simulink model "VCU_SW"  (R2020b)
settings: Solver=FixedStepDiscrete  StartTime=0.0  StopTime=inf  FixedStep=1e-2  RelTol=1e-3
PreLoadFcn:
  | RTWConfigurationCB('preloadfcn', bdroot);
InitFcn:
  | loadvar_ttc500
undefined symbols (not defined in the file): BrkPedalTypes, CabMovModeTypes, cFuseTempSensAcc_X, cFuseTempSensAcc_Y, cFuseTempSensVal_X, cFuseTempSensVal_Y, cTMSTempSensVal_X, cTMSTempSensVal_Y, cTransferCaseSpeedRatio, diag_state, DoorsPositionTypes, dP_filter_Y, DriverOccClassSystemTypes, ErrorValueTypes, fatal_error_callback, IO_ADC_NO_RANGE, LadderStatusTypes, pAnalogCabRotSensAcc, pAnalogCabRotSensMaxVolt, pAnalogCabRotSensMinVolt, pAnalogCabRotSensRange, pAnalogCabRotSensZeroVolt, pBrkActivePress, pCabTiltSensAcc, pCabTiltSensMaxCur, pCabTiltSensMinCur, pDistanceCorrection, pECANManual_BPNEnable, pECANManual_BPNEnabler_Flag, pFilterSensAccRes, pHDirMaxDiffFrq, pHDirSensHighLvl, pHDirSensLowLvl, pMainGearRatio, pMaxFilterSensRes, pMaxFirstPedalSensValue, pMaxFuseTempSensRes, pMaxPressLoss, pMaxPressSensCurrent, pMaxPressValue, pMaxPressValueHydMotAndPump, pMaxPressValueParkDrain, pMaxSecondPedalSensValue, pMaxTempSensVoltage, pMaxTempValue, pMaxTMSTempSensRes, pMinFilterSensRes, pMinFirstPedalSensValue, pMinFuseTempSensRes, pMinPressLoss, pMinPressSensCurrent, pMinPressValue, pMinSecondPedalSensValue, pMinTempSensVoltage, pMinTempValue, pMinTMSTempSensRes, pMotorRingTeethNum, pPedalSensAccuracyPct, pPedalSensAccuracyVolt, pPressLossTreshhold ... (+20)
libraries: TTlibrary x270, canmsglib x127, simulink x88
(part 9 of 17)

== system VCU_SW/OutputLayer/OutputNetwork/OutputEngCAN/SetEngCAN50msec ==
  function : TriggerPort  TriggerType=function-call  VariantControl=Variant
  Bus Selector1 : BusSelector  OutputSignals=ID  OutputAsBus=on
  CANPack_VCU_ECU_TSC1 : canmsglib/CAN Pack  MsgList=(none)  MsgName=VCU_ECU_TSC1  MsgIDType=Extended (29-bit identifier)  MsgIdentifier=201326599  MsgLength=8  Remote=off  ApplyMinMax=off  BusOutput=on  SignalInfo={ 'VCU_ECU_TSC1_ContPurp', '35', '5', 'LE', 'unsigned', 'Standard', '0', '1', '0', '0', '31'; 'VCU_ECU_TSC1_EngOverContMod', '0', '2', 'LE', 'unsigned', 'Standard', '0', '1', '0', '0', '3'; 'VCU_ECU_TSC1_EngReqSpContCond', '2', '2', 'LE', 'unsigned', 'Standard', '0', '1', '0', '0', '3'; 'VCU_ECU_TSC1_EngReqSpSL', '8', '16', 'LE', 'unsigned', 'Standard', '0', '0.125', '0', '0', '8031.875'; 'VCU_ECU_TSC1_EngReqTrqHR', '40', '4', 'LE', 'unsigned', 'Standard', '0', '0.125', '0', '0', '0.875'; 'VCU_ECU_TSC1_EngReqTrqTL', '24', '8', 'LE', 'unsigned', 'Standard', '0', '1', '-125', '-125', '125'; 'VCU_ECU_TSC1_MesChksum', '60', '4', 'LE', 'unsigned', 'Standard', '0', '1', '0', '0', '15'; 'VCU_ECU_TSC1_MessCnt', '56', '4', 'LE', 'unsigned', 'Standard', '0', '1', '0', '0', '15'; 'VCU_ECU_TSC1_OverContModPr', '4', '2', 'LE', 'unsigned', 'Standard', '0', '1', '0', '0', '3'; 'VCU_ECU_TSC1_TransRate', '32', '3', 'LE', 'unsigned', 'Standard', '0', '1', '0', '0', '7' }
      settings: SourceProductBaseCode=ME,XP,VN  DataFormat=manually specified signals
  Constant1 : Constant  Value=uint8(0)
  Data Store Read1 : DataStoreRead  DataStoreName=OutputNetworkData  DataStoreElements=OutputNetworkData.EngCAN.ContPurp#OutputNetworkData.EngCAN.EngOverContMod#OutputNetworkData.EngCAN.EngReqSpContCond#OutputNetworkData.EngCAN.EngReqSpSL#OutputNetworkData.EngCAN.EngReqTrqHR#OutputNetworkData.EngCAN.EngReqTrqTL#OutputNetworkData.EngCAN.MesChksum#OutputNetworkData.EngCAN.MessCnt#OutputNetworkData.EngCAN.OverContModPr#OutputNetworkData.EngCAN.TransRate
  Function-Call Subsystem1 : Subsystem  TreatAsAtomicUnit=on
  Less Than1 : RelationalOperator  Operator=>  OutDataTypeStr=boolean  RndMeth=Simplest
  transmit_vcu_ecu_tsc1 : TTlibrary/CAN/transmit_message_name  channel=IO_CAN_CHANNEL_2  id_format=IO_CAN_EXT_FRAME  retranslation=off  io_error=on  sample_time=-1
      settings: SourceProductName=TT control 500 series
  wires:
  Less Than1/1 -> Function-Call Subsystem1/Enable
  Data Store Read1/2 -> CANPack_VCU_ECU_TSC1/2
  Data Store Read1/5 -> CANPack_VCU_ECU_TSC1/5
  Data Store Read1/1 -> CANPack_VCU_ECU_TSC1/1
  Constant1/1 -> Less Than1/2
  Data Store Read1/9 -> CANPack_VCU_ECU_TSC1/9
  Data Store Read1/8 -> CANPack_VCU_ECU_TSC1/8
  transmit_vcu_ecu_tsc1/1 -> Function-Call Subsystem1/2(error_sts), Less Than1/1  "error_tx_transmit_vcu_ecu_tsc1"
  Data Store Read1/6 -> CANPack_VCU_ECU_TSC1/6
  CANPack_VCU_ECU_TSC1/1 -> Bus Selector1/1, transmit_vcu_ecu_tsc1/1
  Data Store Read1/7 -> CANPack_VCU_ECU_TSC1/7
  Data Store Read1/10 -> CANPack_VCU_ECU_TSC1/10
  Data Store Read1/4 -> CANPack_VCU_ECU_TSC1/4
  Bus Selector1/1 -> Function-Call Subsystem1/1(In1)
  Data Store Read1/3 -> CANPack_VCU_ECU_TSC1/3

== system VCU_SW/OutputLayer/OutputNetwork/OutputHydCAN/SetHydCAN100msec ==
  note: См. outputFcn
  function : TriggerPort  TriggerType=function-call  VariantControl=Variant
  CANPack_hyd_Fluid_temp : canmsglib/CAN Pack  Commented=on  MsgList=(none)  MsgName=VEH_FLUID_TEMP  MsgIDType=Extended (29-bit identifier)  MsgIdentifier=419326202  MsgLength=1  Remote=off  ApplyMinMax=off  BusOutput=on  SignalInfo={ 'FluidTemp', '0', '8', 'LE', 'signed', 'Standard', '0', '1', '40', '-40', '120' }
      settings: SourceProductBaseCode=ME,XP,VN  DataFormat=manually specified signals
  Cabine1stLeftHydCylValve : Subsystem
  Cabine2ndRightHydCylValve : Subsystem
  CabineTurningValve : Subsystem
  Data Store Read : DataStoreRead  Commented=on  DataStoreName=OutputNetworkData  DataStoreElements=OutputNetworkData.HydCAN.fluidTemp
  Terminator : Terminator  Commented=on
  transmit_message_hyd_fluid_temp : TTlibrary/CAN/transmit_message_name  Commented=on  channel=IO_CAN_CHANNEL_0  id_format=IO_CAN_EXT_FRAME  retranslation=off  io_error=on  sample_time=-1
      settings: SourceProductName=TT control 500 series
  wires:
  transmit_message_hyd_fluid_temp/1 -> Terminator/1  "error_tx_transmit_message_hyd_fluid_temp"
  CANPack_hyd_Fluid_temp/1 -> transmit_message_hyd_fluid_temp/1
  Data Store Read/1 -> CANPack_hyd_Fluid_temp/1

== system VCU_SW/OutputLayer/OutputNetwork/OutputStrCAN/SetStrCAN100msec ==
  note: См. outputFcn
  function : TriggerPort  TriggerType=function-call  VariantControl=Variant
  CANPack_Str_Fluid_temp : canmsglib/CAN Pack  Commented=on  MsgList=(none)  MsgName=VEH_FLUID_TEMP  MsgIDType=Extended (29-bit identifier)  MsgIdentifier=419326202  MsgLength=1  Remote=off  ApplyMinMax=off  BusOutput=on  SignalInfo={ 'FluidTemp', '0', '8', 'LE', 'signed', 'Standard', '0', '1', '40', '-40', '120' }
      settings: SourceProductBaseCode=ME,XP,VN  DataFormat=manually specified signals
  CANPack_VLVCMD_STR1 : canmsglib/CAN Pack  MsgList=(none)  MsgName=VLVCMD_STR1  MsgIDType=Extended (29-bit identifier)  MsgIdentifier=217985274  MsgLength=3  Remote=off  ApplyMinMax=off  BusOutput=on  SignalInfo={ 'FailSafeModeCmdStr1', '22', '2', 'LE', 'unsigned', 'Standard', '0', '1', '0', '0', '3'; 'PortFlowCmdStr1', '0', '8', 'LE', 'unsigned', 'Standard', '0', '0.4', '0', '0', '100'; 'ValveStateStr1', '16', '4', 'LE', 'unsigned', 'Standard', '0', '1', '0', '0', '15' }
      settings: SourceProductBaseCode=ME,XP,VN  DataFormat=manually specified signals
  Data Store Read : DataStoreRead  Commented=on  DataStoreName=OutputNetworkData  DataStoreElements=OutputNetworkData.StrCAN.fluidTemp
  Data Store Read1 : DataStoreRead  DataStoreName=OutputNetworkData  DataStoreElements=OutputNetworkData.StrCAN.failSafeModeCmdStr1#OutputNetworkData.StrCAN.portFlowCmdStr1#OutputNetworkData.StrCAN.valveStateStr1
  Terminator : Terminator  Commented=on
  Terminator1 : Terminator
  transmit_message_str_fluid_temp : TTlibrary/CAN/transmit_message_name  Commented=on  channel=IO_CAN_CHANNEL_3  id_format=IO_CAN_EXT_FRAME  retranslation=off  io_error=on  sample_time=-1
      settings: SourceProductName=TT control 500 series
  transmit_message_vlvcmd_str1 : TTlibrary/CAN/transmit_message_name  channel=IO_CAN_CHANNEL_3  id_format=IO_CAN_EXT_FRAME  retranslation=off  io_error=on  sample_time=-1
      settings: SourceProductName=TT control 500 series
  wires:
  CANPack_Str_Fluid_temp/1 -> transmit_message_str_fluid_temp/1
  transmit_message_str_fluid_temp/1 -> Terminator/1  "error_tx_transmit_message_str_fluid_temp"
  Data Store Read/1 -> CANPack_Str_Fluid_temp/1
  Data Store Read1/1 -> CANPack_VLVCMD_STR1/1
  transmit_message_vlvcmd_str1/1 -> Terminator1/1  "error_tx_transmit_message_vlvcmd_str1"
  CANPack_VLVCMD_STR1/1 -> transmit_message_vlvcmd_str1/1
  Data Store Read1/2 -> CANPack_VLVCMD_STR1/2
  Data Store Read1/3 -> CANPack_VLVCMD_STR1/3

== system VCU_SW/logSignal/getListData/pageHighvoltageAppData/getListDataII1 ==
  getListDataII1 : TriggerPort  TriggerType=function-call  IsSimulinkFunction=on  FunctionName=getListDataII1  FunctionVisibility=scoped  VariantControl=(inherit)
  Constant : Constant  Value=uint8(5)
  Data Store Read1 : DataStoreRead  DataStoreName=sBmsCounter
  Data Store Read2 : DataStoreRead  DataStoreName=sChargeStopSignal
  Data Store Read3 : DataStoreRead  DataStoreName=sStopAll
  Data Store Read4 : DataStoreRead  DataStoreName=sBmsLocalState
  Demux11 : Demux  Outputs=2
  Function Caller : FunctionCaller  FunctionPrototype=data = getListData.splitIntoTwoBytes(value)  InputArgumentSpecifications=<Enter example>  OutputArgumentSpecifications=<Enter example>
  Ground : Ground
  Mux : Mux  Inputs=7
  data : ArgOut  DisableCoverage=on  OutDataTypeStr=uint8  PortDimensions=[1,7]  ArgumentName=data
  len : ArgOut  Port=2  OutDataTypeStr=uint8  ArgumentName=len
  wires:
  Data Store Read2/1 -> Mux/4
  Data Store Read3/1 -> Mux/5
  Demux11/2 -> Mux/3
  Data Store Read4/1 -> Mux/1
  Demux11/1 -> Mux/2
  Mux/1 -> data/1
  Constant/1 -> len/1
  Function Caller/1 -> Demux11/1
  Data Store Read1/1 -> Function Caller/1
  Ground/1 -> Mux/6, Mux/7

== system VCU_SW/logSignal/getListData/pageHighvoltageAppData/getListDataII10 ==
  getListDataII10 : TriggerPort  TriggerType=function-call  IsSimulinkFunction=on  FunctionName=getListDataII10  FunctionVisibility=scoped  VariantControl=(inherit)
  Constant : Constant  Value=uint8(4)
  Data Store Read1 : DataStoreRead  DataStoreName=sB5_modes_1
  Data Store Read2 : DataStoreRead  DataStoreName=sB5_mode_1
  Data Store Read5 : DataStoreRead  DataStoreName=sB5_ChargeMode
  Data Store Read6 : DataStoreRead  DataStoreName=sB5_power
  Ground : Ground
  Mux : Mux  Inputs=7
  data : ArgOut  DisableCoverage=on  OutDataTypeStr=uint8  PortDimensions=[1,7]  ArgumentName=data
  len : ArgOut  Port=2  OutDataTypeStr=uint8  ArgumentName=len
  wires:
  Mux/1 -> data/1
  Constant/1 -> len/1
  Data Store Read5/1 -> Mux/4
  Data Store Read6/1 -> Mux/3
  Data Store Read2/1 -> Mux/1
  Data Store Read1/1 -> Mux/2
  Ground/1 -> Mux/7, Mux/6, Mux/5

== system VCU_SW/logSignal/getListData/pageHighvoltageAppData/getListDataII11 ==
  getListDataII11 : TriggerPort  TriggerType=function-call  IsSimulinkFunction=on  FunctionName=getListDataII11  FunctionVisibility=scoped  VariantControl=(inherit)
  Constant : Constant  Value=uint8(5)
  Data Store Read1 : DataStoreRead  DataStoreName=sPlugUnlockPerm
  Data Store Read2 : DataStoreRead  DataStoreName=sChargeLocalState
  Data Store Read3 : DataStoreRead  DataStoreName=sChargePerm
  Data Store Read4 : DataStoreRead  DataStoreName=sPlugLockPerm
  Data Store Read5 : DataStoreRead  DataStoreName=sPrechargeComplete
  Ground : Ground
  Mux : Mux  Inputs=7
  data : ArgOut  DisableCoverage=on  OutDataTypeStr=uint8  PortDimensions=[1,7]  ArgumentName=data
  len : ArgOut  Port=2  OutDataTypeStr=uint8  ArgumentName=len
  wires:
  Mux/1 -> data/1
  Constant/1 -> len/1
  Data Store Read4/1 -> Mux/1
  Data Store Read1/1 -> Mux/2
  Data Store Read3/1 -> Mux/3
  Data Store Read2/1 -> Mux/4
  Data Store Read5/1 -> Mux/5
  Ground/1 -> Mux/6, Mux/7

== system VCU_SW/logSignal/getListData/pageHighvoltageAppData/getListDataII12 ==
  note: -32767 to 32767
  getListDataII12 : TriggerPort  TriggerType=function-call  IsSimulinkFunction=on  FunctionName=getListDataII12  FunctionVisibility=scoped  VariantControl=(inherit)
  Constant : Constant  Value=uint8(6)
  Data Store Read1 : DataStoreRead  DataStoreName=sAimTrq
  Data Store Read2 : DataStoreRead  DataStoreName=sT15GroupStt
  Data Store Read4 : DataStoreRead  DataStoreName=sInvLocalState
  Data Store Read5 : DataStoreRead  DataStoreName=sCurStepInv
  Data Type Conversion : DataTypeConversion  OutDataTypeStr=int32
  Data Type Conversion1 : DataTypeConversion  OutDataTypeStr=uint16
  Data Type Conversion2 : DataTypeConversion  OutDataTypeStr=int32
  Data Type Conversion3 : DataTypeConversion  OutDataTypeStr=uint16
  Demux1 : Demux  Outputs=2
  Demux11 : Demux  Outputs=2
  Function Caller : FunctionCaller  FunctionPrototype=data = getListData.splitIntoTwoBytes(value)  InputArgumentSpecifications=<Enter example>  OutputArgumentSpecifications=<Enter example>
  Function Caller1 : FunctionCaller  FunctionPrototype=data = getListData.splitIntoTwoBytes(value)  InputArgumentSpecifications=<Enter example>  OutputArgumentSpecifications=<Enter example>
  Ground : Ground
  Mux : Mux  Inputs=7
  Sum2 : Sum  Inputs=++|
  Sum3 : Sum  Inputs=|++
  offset : Constant  Value=int32(32767)
  data : ArgOut  DisableCoverage=on  OutDataTypeStr=uint8  PortDimensions=[1,7]  ArgumentName=data
  len : ArgOut  Port=2  OutDataTypeStr=uint8  ArgumentName=len
  wires:
  Ground/1 -> Mux/7
  Constant/1 -> len/1
  Mux/1 -> data/1
  Demux11/2 -> Mux/3
  Data Store Read1/1 -> Data Type Conversion2/1
  Function Caller/1 -> Demux11/1
  Demux11/1 -> Mux/2
  Data Store Read4/1 -> Mux/1
  Function Caller1/1 -> Demux1/1
  Demux1/2 -> Mux/5
  Demux1/1 -> Mux/4
  Data Store Read2/1 -> Mux/6
  Data Store Read5/1 -> Data Type Conversion/1
  Sum2/1 -> Data Type Conversion1/1
  Data Type Conversion1/1 -> Function Caller1/1
  Data Type Conversion/1 -> Sum2/2
  offset/1 -> Sum2/1, Sum3/2
  Sum3/1 -> Data Type Conversion3/1
  Data Type Conversion2/1 -> Sum3/1
  Data Type Conversion3/1 -> Function Caller/1

== system VCU_SW/logSignal/getListData/pageHighvoltageAppData/getListDataII2 ==
  getListDataII2 : TriggerPort  TriggerType=function-call  IsSimulinkFunction=on  FunctionName=getListDataII2  FunctionVisibility=scoped  VariantControl=(inherit)
  Constant : Constant  Value=uint8(4)
  Data Store Read1 : DataStoreRead  DataStoreName=sPermissibleChargeCurrent
  Data Store Read2 : DataStoreRead  DataStoreName=sPermissibleChargeVoltage
  Demux1 : Demux  Outputs=2
  Demux11 : Demux  Outputs=2
  Function Caller : FunctionCaller  FunctionPrototype=data = getListData.splitIntoTwoBytes(value)  InputArgumentSpecifications=<Enter example>  OutputArgumentSpecifications=<Enter example>
  Function Caller1 : FunctionCaller  FunctionPrototype=data = getListData.splitIntoTwoBytes(value)  InputArgumentSpecifications=<Enter example>  OutputArgumentSpecifications=<Enter example>
  Ground : Ground
  Mux : Mux  Inputs=7
  data : ArgOut  DisableCoverage=on  OutDataTypeStr=uint8  PortDimensions=[1,7]  ArgumentName=data
  len : ArgOut  Port=2  OutDataTypeStr=uint8  ArgumentName=len
  wires:
  Mux/1 -> data/1
  Constant/1 -> len/1
  Function Caller/1 -> Demux11/1
  Demux11/1 -> Mux/1
  Data Store Read1/1 -> Function Caller/1
  Demux11/2 -> Mux/2
  Demux1/1 -> Mux/3
  Function Caller1/1 -> Demux1/1
  Data Store Read2/1 -> Function Caller1/1
  Demux1/2 -> Mux/4
  Ground/1 -> Mux/5, Mux/6, Mux/7

== system VCU_SW/logSignal/getListData/pageHighvoltageAppData/getListDataII3 ==
  getListDataII3 : TriggerPort  TriggerType=function-call  IsSimulinkFunction=on  FunctionName=getListDataII3  FunctionVisibility=scoped  VariantControl=(inherit)
  Constant : Constant  Value=uint8(7)
  Data Store Read1 : DataStoreRead  DataStoreName=sCompressorPwm
  Data Store Read2 : DataStoreRead  DataStoreName=sTmsCounter
  Data Store Read3 : DataStoreRead  DataStoreName=sPumpPwm
  Data Store Read4 : DataStoreRead  DataStoreName=sFanControl
  Data Store Read5 : DataStoreRead  DataStoreName=sTmsLocalState
  Data Store Read6 : DataStoreRead  DataStoreName=sTmsCircleSelected
  Demux1 : Demux  Outputs=2
  Function Caller1 : FunctionCaller  FunctionPrototype=data = getListData.splitIntoTwoBytes(value)  InputArgumentSpecifications=<Enter example>  OutputArgumentSpecifications=<Enter example>
  Mux : Mux  Inputs=7
  data : ArgOut  DisableCoverage=on  OutDataTypeStr=uint8  PortDimensions=[1,7]  ArgumentName=data
  len : ArgOut  Port=2  OutDataTypeStr=uint8  ArgumentName=len
  wires:
  Mux/1 -> data/1
  Constant/1 -> len/1
  Function Caller1/1 -> Demux1/1
  Data Store Read2/1 -> Function Caller1/1
  Demux1/1 -> Mux/6
  Demux1/2 -> Mux/7
  Data Store Read1/1 -> Mux/1
  Data Store Read3/1 -> Mux/2
  Data Store Read4/1 -> Mux/3
  Data Store Read5/1 -> Mux/4
  Data Store Read6/1 -> Mux/5

== system VCU_SW/logSignal/getListData/pageHighvoltageAppData/getListDataII4 ==
  getListDataII4 : TriggerPort  TriggerType=function-call  IsSimulinkFunction=on  FunctionName=getListDataII4  FunctionVisibility=scoped  VariantControl=(inherit)
  Constant : Constant  Value=uint8(7)
  Data Store Read1 : DataStoreRead  DataStoreName=sCompressorCounter
  Data Store Read2 : DataStoreRead  DataStoreName=sValveControl
  Data Store Read3 : DataStoreRead  DataStoreName=sPreviousState
  Data Store Read4 : DataStoreRead  DataStoreName=sHeaterEnable
  Data Store Read5 : DataStoreRead  DataStoreName=sHeaterPowerControl
  Data Store Read6 : DataStoreRead  DataStoreName=sCompressorStart
  Demux11 : Demux  Outputs=2
  Function Caller : FunctionCaller  FunctionPrototype=data = getListData.splitIntoTwoBytes(value)  InputArgumentSpecifications=<Enter example>  OutputArgumentSpecifications=<Enter example>
  Mux : Mux  Inputs=7
  data : ArgOut  DisableCoverage=on  OutDataTypeStr=uint8  PortDimensions=[1,7]  ArgumentName=data
  len : ArgOut  Port=2  OutDataTypeStr=uint8  ArgumentName=len
  wires:
  Mux/1 -> data/1
  Constant/1 -> len/1
  Function Caller/1 -> Demux11/1
  Demux11/1 -> Mux/1
  Data Store Read1/1 -> Function Caller/1
  Demux11/2 -> Mux/2
  Data Store Read3/1 -> Mux/6
  Data Store Read2/1 -> Mux/7
  Data Store Read4/1 -> Mux/5
  Data Store Read5/1 -> Mux/4
  Data Store Read6/1 -> Mux/3

== system VCU_SW/logSignal/getListData/pageHighvoltageAppData/getListDataII5 ==
  getListDataII5 : TriggerPort  TriggerType=function-call  IsSimulinkFunction=on  FunctionName=getListDataII5  FunctionVisibility=scoped  VariantControl=(inherit)
  Constant : Constant  Value=uint8(7)
  Data Store Read1 : DataStoreRead  DataStoreName=sSelfCircCounter
  Data Store Read2 : DataStoreRead  DataStoreName=sCompressoSecondCircleEx
  Data Store Read3 : DataStoreRead  DataStoreName=sCompressorStartEx
  Data Store Read4 : DataStoreRead  DataStoreName=sCompressorOffEx
  Data Store Read5 : DataStoreRead  DataStoreName=sPumpSecondCircleEx
  Data Store Read6 : DataStoreRead  DataStoreName=sPumpOffEx
  Demux11 : Demux  Outputs=2
  Function Caller : FunctionCaller  FunctionPrototype=data = getListData.splitIntoTwoBytes(value)  InputArgumentSpecifications=<Enter example>  OutputArgumentSpecifications=<Enter example>
  Mux : Mux  Inputs=7
  data : ArgOut  DisableCoverage=on  OutDataTypeStr=uint8  PortDimensions=[1,7]  ArgumentName=data
  len : ArgOut  Port=2  OutDataTypeStr=uint8  ArgumentName=len
  wires:
  Mux/1 -> data/1
  Constant/1 -> len/1
  Function Caller/1 -> Demux11/1
  Demux11/1 -> Mux/1
  Data Store Read1/1 -> Function Caller/1
  Demux11/2 -> Mux/2
  Data Store Read2/1 -> Mux/7
  Data Store Read3/1 -> Mux/6
  Data Store Read4/1 -> Mux/5
  Data Store Read5/1 -> Mux/4
  Data Store Read6/1 -> Mux/3

== system VCU_SW/logSignal/getListData/pageHighvoltageAppData/getListDataII6 ==
  getListDataII6 : TriggerPort  TriggerType=function-call  IsSimulinkFunction=on  FunctionName=getListDataII6  FunctionVisibility=scoped  VariantControl=(inherit)
  Constant : Constant  Value=uint8(7)
  Data Store Read1 : DataStoreRead  DataStoreName=sEproCurrent
  Data Store Read2 : DataStoreRead  DataStoreName=sHeaterSecondCircleEx
  Data Store Read3 : DataStoreRead  DataStoreName=sHeaterTempEx
  Data Store Read4 : DataStoreRead  DataStoreName=sHeaterOffEx
  Data Store Read5 : DataStoreRead  DataStoreName=sEproStartCommand
  Data Store Read6 : DataStoreRead  DataStoreName=sEproPower
  Demux11 : Demux  Outputs=2
  Function Caller : FunctionCaller  FunctionPrototype=data = getListData.splitIntoTwoBytes(value)  InputArgumentSpecifications=<Enter example>  OutputArgumentSpecifications=<Enter example>
  Mux : Mux  Inputs=7
  data : ArgOut  DisableCoverage=on  OutDataTypeStr=uint8  PortDimensions=[1,7]  ArgumentName=data
  len : ArgOut  Port=2  OutDataTypeStr=uint8  ArgumentName=len
  wires:
  Mux/1 -> data/1
  Constant/1 -> len/1
  Data Store Read3/1 -> Mux/2
  Data Store Read4/1 -> Mux/1
  Data Store Read2/1 -> Mux/3
  Demux11/2 -> Mux/6
  Data Store Read1/1 -> Function Caller/1
  Function Caller/1 -> Demux11/1
  Demux11/1 -> Mux/5
  Data Store Read5/1 -> Mux/7
  Data Store Read6/1 -> Mux/4

== system VCU_SW/logSignal/getListData/pageHighvoltageAppData/getListDataII7 ==
  getListDataII7 : TriggerPort  TriggerType=function-call  IsSimulinkFunction=on  FunctionName=getListDataII7  FunctionVisibility=scoped  VariantControl=(inherit)
  Constant : Constant  Value=uint8(6)
  Data Store Read1 : DataStoreRead  DataStoreName=sPosIsolationResistence
  Data Store Read2 : DataStoreRead  DataStoreName=sNegIsolationResistence
  Data Store Read3 : DataStoreRead  DataStoreName=sMaxCellVoltage
  Demux1 : Demux  Outputs=2
  Demux11 : Demux  Outputs=2
  Demux2 : Demux  Outputs=2
  Function Caller : FunctionCaller  FunctionPrototype=data = getListData.splitIntoTwoBytes(value)  InputArgumentSpecifications=<Enter example>  OutputArgumentSpecifications=<Enter example>
  Function Caller1 : FunctionCaller  FunctionPrototype=data = getListData.splitIntoTwoBytes(value)  InputArgumentSpecifications=<Enter example>  OutputArgumentSpecifications=<Enter example>
  Function Caller2 : FunctionCaller  FunctionPrototype=data = getListData.splitIntoTwoBytes(value)  InputArgumentSpecifications=<Enter example>  OutputArgumentSpecifications=<Enter example>
  Ground : Ground
  Mux : Mux  Inputs=7
  data : ArgOut  DisableCoverage=on  OutDataTypeStr=uint8  PortDimensions=[1,7]  ArgumentName=data
  len : ArgOut  Port=2  OutDataTypeStr=uint8  ArgumentName=len
  wires:
  Demux11/2 -> Mux/2
  Data Store Read1/1 -> Function Caller/1
  Demux11/1 -> Mux/1
  Function Caller/1 -> Demux11/1
  Constant/1 -> len/1
  Mux/1 -> data/1
  Function Caller1/1 -> Demux1/1
  Demux1/1 -> Mux/3
  Data Store Read2/1 -> Function Caller1/1
  Demux1/2 -> Mux/4
  Demux2/2 -> Mux/6
  Data Store Read3/1 -> Function Caller2/1
  Demux2/1 -> Mux/5
  Function Caller2/1 -> Demux2/1
  Ground/1 -> Mux/7

== system VCU_SW/logSignal/getListData/pageHighvoltageAppData/getListDataII8 ==
  getListDataII8 : TriggerPort  TriggerType=function-call  IsSimulinkFunction=on  FunctionName=getListDataII8  FunctionVisibility=scoped  VariantControl=(inherit)
  Constant : Constant  Value=uint8(6)
  Data Store Read1 : DataStoreRead  DataStoreName=sMinCellVoltage
  Data Store Read2 : DataStoreRead  DataStoreName=sMaxBatTemp
  Data Store Read3 : DataStoreRead  DataStoreName=sMinBatTemp
  Demux1 : Demux  Outputs=2
  Demux11 : Demux  Outputs=2
  Demux2 : Demux  Outputs=2
  Function Caller : FunctionCaller  FunctionPrototype=data = getListData.splitIntoTwoBytes(value)  InputArgumentSpecifications=<Enter example>  OutputArgumentSpecifications=<Enter example>
  Function Caller1 : FunctionCaller  FunctionPrototype=data = getListData.splitIntoTwoBytes(value)  InputArgumentSpecifications=<Enter example>  OutputArgumentSpecifications=<Enter example>
  Function Caller2 : FunctionCaller  FunctionPrototype=data = getListData.splitIntoTwoBytes(value)  InputArgumentSpecifications=<Enter example>  OutputArgumentSpecifications=<Enter example>
  Ground : Ground
  Mux : Mux  Inputs=7
  data : ArgOut  DisableCoverage=on  OutDataTypeStr=uint8  PortDimensions=[1,7]  ArgumentName=data
  len : ArgOut  Port=2  OutDataTypeStr=uint8  ArgumentName=len
  wires:
  Mux/1 -> data/1
  Constant/1 -> len/1
  Function Caller/1 -> Demux11/1
  Demux11/1 -> Mux/1
  Data Store Read1/1 -> Function Caller/1
  Demux11/2 -> Mux/2
  Demux1/2 -> Mux/4
  Data Store Read2/1 -> Function Caller1/1
  Demux1/1 -> Mux/3
  Function Caller1/1 -> Demux1/1
  Function Caller2/1 -> Demux2/1
  Demux2/2 -> Mux/6
  Demux2/1 -> Mux/5
  Ground/1 -> Mux/7
  Data Store Read3/1 -> Function Caller2/1

== system VCU_SW/logSignal/getListData/pageHighvoltageAppData/getListDataII9 ==
  getListDataII9 : TriggerPort  TriggerType=function-call  IsSimulinkFunction=on  FunctionName=getListDataII9  FunctionVisibility=scoped  VariantControl=(inherit)
  Constant : Constant  Value=uint8(6)
  Data Store Read1 : DataStoreRead  DataStoreName=sTotalVoltage
  Data Store Read2 : DataStoreRead  DataStoreName=sMaxCellVoltTemp
  Data Store Read3 : DataStoreRead  DataStoreName=sMinCellVoltTemp
  Data Store Read4 : DataStoreRead  DataStoreName=sSettingTargetWaterTemp
  Data Store Read5 : DataStoreRead  DataStoreName=sAverageBatTemp
  Demux11 : Demux  Outputs=2
  Function Caller : FunctionCaller  FunctionPrototype=data = getListData.splitIntoTwoBytes(value)  InputArgumentSpecifications=<Enter example>  OutputArgumentSpecifications=<Enter example>
  Ground : Ground
  Mux : Mux  Inputs=7
  data : ArgOut  DisableCoverage=on  OutDataTypeStr=uint8  PortDimensions=[1,7]  ArgumentName=data
  len : ArgOut  Port=2  OutDataTypeStr=uint8  ArgumentName=len
  wires:
  Data Store Read1/1 -> Function Caller/1
  Function Caller/1 -> Demux11/1
  Constant/1 -> len/1
  Mux/1 -> data/1
  Demux11/1 -> Mux/3
  Demux11/2 -> Mux/4
  Data Store Read3/1 -> Mux/2
  Data Store Read2/1 -> Mux/1
  Data Store Read4/1 -> Mux/5
  Data Store Read5/1 -> Mux/6
  Ground/1 -> Mux/7

== system VCU_SW/logSignal/getListData/pageOutputRawData/getListDataOI1 ==
  getListDataOI1 : TriggerPort  TriggerType=function-call  IsSimulinkFunction=on  FunctionName=getListDataOI1  FunctionVisibility=scoped  VariantControl=(inherit)
  Data Store Read2 : DataStoreRead  DataStoreName=sCoolSensSup
  Data Store Read3 : DataStoreRead  DataStoreName=sOnBrdChrgTermSttSup
  Data Store Read4 : DataStoreRead  DataStoreName=sHVILSup
  Data Store Read5 : DataStoreRead  DataStoreName=sOnBrdFastChrgSup
  Data Store Read6 : DataStoreRead  DataStoreName=sPressSensSup
  Data Store Read7 : DataStoreRead  DataStoreName=sGearboxSensSup
  Data Store Read8 : DataStoreRead  DataStoreName=sACDCChrgConvSwt
  Mux : Mux  Inputs=7
  data : ArgOut  DisableCoverage=on  OutDataTypeStr=uint8  PortDimensions=[1,7]  ArgumentName=data
  wires:
  Mux/1 -> data/1
  Data Store Read2/1 -> Mux/7
  Data Store Read3/1 -> Mux/6
  Data Store Read8/1 -> Mux/1
  Data Store Read4/1 -> Mux/5
  Data Store Read7/1 -> Mux/2
  Data Store Read5/1 -> Mux/4
  Data Store Read6/1 -> Mux/3

== system VCU_SW/logSignal/getListData/pageOutputRawData/getListDataOI2 ==
  getListDataOI2 : TriggerPort  TriggerType=function-call  IsSimulinkFunction=on  FunctionName=getListDataOI2  FunctionVisibility=scoped  VariantControl=(inherit)
  Data Store Read : DataStoreRead  DataStoreName=sCapsSup
  Data Store Read1 : DataStoreRead  DataStoreName=sPumpFlowSetPnt
  Data Store Read12 : DataStoreRead  DataStoreName=sTMSComprSetPnt
  Data Store Read13 : DataStoreRead  DataStoreName=sCircPumpSetPnt
  Demux : Demux  Outputs=2
  Demux1 : Demux  Outputs=2
  Demux2 : Demux  Outputs=2
  Function Caller3 : FunctionCaller  FunctionPrototype=data = getListData.splitIntoTwoBytes(value)  InputArgumentSpecifications=<Enter example>  OutputArgumentSpecifications=<Enter example>
  Function Caller4 : FunctionCaller  FunctionPrototype=data = getListData.splitIntoTwoBytes(value)  InputArgumentSpecifications=<Enter example>  OutputArgumentSpecifications=<Enter example>
  Function Caller5 : FunctionCaller  FunctionPrototype=data = getListData.splitIntoTwoBytes(value)  InputArgumentSpecifications=<Enter example>  OutputArgumentSpecifications=<Enter example>
  Mux1 : Mux  Inputs=7
  data : ArgOut  DisableCoverage=on  OutDataTypeStr=uint8  PortDimensions=[1,7]  ArgumentName=data
  wires:
  Mux1/1 -> data/1
  Data Store Read12/1 -> Function Caller4/1
  Demux1/1 -> Mux1/3
  Demux/2 -> Mux1/2
  Demux2/1 -> Mux1/5
  Demux/1 -> Mux1/1
  Data Store Read13/1 -> Function Caller5/1
  Demux2/2 -> Mux1/6
  Function Caller3/1 -> Demux/1
  Data Store Read1/1 -> Function Caller3/1
  Data Store Read/1 -> Mux1/7
  Demux1/2 -> Mux1/4
  Function Caller4/1 -> Demux1/1
  Function Caller5/1 -> Demux2/1

== system VCU_SW/logSignal/getListData/pageOutputRawData/getListDataOI3 ==
  getListDataOI3 : TriggerPort  TriggerType=function-call  IsSimulinkFunction=on  FunctionName=getListDataOI3  FunctionVisibility=scoped  VariantControl=(inherit)
  Data Store Read10 : DataStoreRead  DataStoreName=sSecondGearVlvSetPnt
  Data Store Read11 : DataStoreRead  DataStoreName=sRemBrkVlvSetPnt
  Data Store Read9 : DataStoreRead  DataStoreName=sFirstGearVlvSetPnt
  Demux3 : Demux  Outputs=2
  Demux4 : Demux  Outputs=2
  Demux5 : Demux  Outputs=2
  Function Caller : FunctionCaller  FunctionPrototype=data = getListData.splitIntoTwoBytes(value)  InputArgumentSpecifications=<Enter example>  OutputArgumentSpecifications=<Enter example>
  Function Caller1 : FunctionCaller  FunctionPrototype=data = getListData.splitIntoTwoBytes(value)  InputArgumentSpecifications=<Enter example>  OutputArgumentSpecifications=<Enter example>
  Function Caller2 : FunctionCaller  FunctionPrototype=data = getListData.splitIntoTwoBytes(value)  InputArgumentSpecifications=<Enter example>  OutputArgumentSpecifications=<Enter example>
  Ground : Ground
  Mux2 : Mux  Inputs=7
  data : ArgOut  DisableCoverage=on  OutDataTypeStr=uint8  PortDimensions=[1,7]  ArgumentName=data
  wires:
  Function Caller1/1 -> Demux4/1
  Function Caller2/1 -> Demux5/1
  Demux4/2 -> Mux2/4
  Demux3/2 -> Mux2/2
  Demux5/1 -> Mux2/5
  Demux3/1 -> Mux2/1
  Demux4/1 -> Mux2/3
  Data Store Read9/1 -> Function Caller/1
  Data Store Read10/1 -> Function Caller1/1
  Ground/1 -> Mux2/7
  Function Caller/1 -> Demux3/1
  Demux5/2 -> Mux2/6
  Data Store Read11/1 -> Function Caller2/1
  Mux2/1 -> data/1

== system VCU_SW/logSignal/getListData/pageRawInput/getListDataII1 ==
  getListDataII1 : TriggerPort  TriggerType=function-call  IsSimulinkFunction=on  FunctionName=getListDataII1  FunctionVisibility=scoped  VariantControl=(inherit)
  Constant : Constant  Value=uint8(7)
  Data Store Read1 : DataStoreRead  DataStoreName=sHVILSup
  Data Store Read2 : DataStoreRead  DataStoreName=sPrechargeCtrlStt
  Data Store Read3 : DataStoreRead  DataStoreName=sDCDCEmergGND
  Data Store Read4 : DataStoreRead  DataStoreName=sACChrgSupTermStt
  Data Store Read5 : DataStoreRead  DataStoreName=sACChrgGndTermStt
  Data Store Read6 : DataStoreRead  DataStoreName=sDCChrgSupTermStt
  Data Store Read7 : DataStoreRead  DataStoreName=sDCChrgGndTermStt
  Mux : Mux  Inputs=7
  data : ArgOut  DisableCoverage=on  OutDataTypeStr=uint8  PortDimensions=[1,7]  ArgumentName=data
  len : ArgOut  Port=2  OutDataTypeStr=uint8  ArgumentName=len
  wires:
  Data Store Read5/1 -> Mux/4
  Data Store Read2/1 -> Mux/7
  Data Store Read3/1 -> Mux/5
  Data Store Read7/1 -> Mux/3
  Data Store Read4/1 -> Mux/1
  Data Store Read6/1 -> Mux/2
  Data Store Read1/1 -> Mux/6
  Mux/1 -> data/1
  Constant/1 -> len/1

== system VCU_SW/logSignal/getListData/pageRawInput/getListDataII2 ==
  getListDataII2 : TriggerPort  TriggerType=function-call  IsSimulinkFunction=on  FunctionName=getListDataII2  FunctionVisibility=scoped  VariantControl=(inherit)
  Constant : Constant  Value=uint8(7)
  Data Store Read : DataStoreRead  DataStoreName=sGlobalSupTermStt
  Data Store Read10 : DataStoreRead  DataStoreName=sFrontCargoWeight
  Data Store Read11 : DataStoreRead  DataStoreName=sRearCargoWeight
  Data Store Read14 : DataStoreRead  DataStoreName=sGearboxOilState
  Demux : Demux  Outputs=2
  Demux1 : Demux  Outputs=2
  Demux2 : Demux  Outputs=2
  Function Caller : FunctionCaller  FunctionPrototype=data = getListData.splitIntoTwoBytes(value)  InputArgumentSpecifications=<Enter example>  OutputArgumentSpecifications=<Enter example>
  Function Caller13 : FunctionCaller  FunctionPrototype=data = getListData.splitIntoTwoBytes(value)  InputArgumentSpecifications=<Enter example>  OutputArgumentSpecifications=<Enter example>
  Function Caller14 : FunctionCaller  FunctionPrototype=data = getListData.splitIntoTwoBytes(value)  InputArgumentSpecifications=<Enter example>  OutputArgumentSpecifications=<Enter example>
  Mux1 : Mux  Inputs=7
  data : ArgOut  DisableCoverage=on  OutDataTypeStr=uint8  PortDimensions=[1,7]  ArgumentName=data
  len : ArgOut  Port=2  OutDataTypeStr=uint8  ArgumentName=len
  wires:
  Data Store Read/1 -> Mux1/7
  Data Store Read14/1 -> Function Caller/1
  Demux2/2 -> Mux1/6
  Demux2/1 -> Mux1/5
  Demux/2 -> Mux1/2
  Data Store Read10/1 -> Function Caller13/1
  Demux/1 -> Mux1/1
  Function Caller/1 -> Demux/1
  Function Caller13/1 -> Demux1/1
  Demux1/1 -> Mux1/3
  Demux1/2 -> Mux1/4
  Function Caller14/1 -> Demux2/1
  Data Store Read11/1 -> Function Caller14/1
  Mux1/1 -> data/1
  Constant/1 -> len/1

== system VCU_SW/logSignal/getListData/pageRawInput/getListDataII3 ==
  getListDataII3 : TriggerPort  TriggerType=function-call  IsSimulinkFunction=on  FunctionName=getListDataII3  FunctionVisibility=scoped  VariantControl=(inherit)
  Constant : Constant  Value=uint8(6)
  Data Store Read12 : DataStoreRead  DataStoreName=sTMSTempInput
  Data Store Read17 : DataStoreRead  DataStoreName=sPumpFlowCur
  Demux3 : Demux
  Demux4 : Demux  Outputs=2
  Function Caller1 : FunctionCaller  FunctionPrototype=data = getListData.splitIntoFourBytes(value)  InputArgumentSpecifications=<Enter example>  OutputArgumentSpecifications=<Enter example>
  Function Caller2 : FunctionCaller  FunctionPrototype=data = getListData.splitIntoTwoBytes(value)  InputArgumentSpecifications=<Enter example>  OutputArgumentSpecifications=<Enter example>
  Ground : Ground
  Mux2 : Mux  Inputs=7
  data : ArgOut  DisableCoverage=on  OutDataTypeStr=uint8  PortDimensions=[1,7]  ArgumentName=data
  len : ArgOut  Port=2  OutDataTypeStr=uint8  ArgumentName=len
  wires:
  Demux4/2 -> Mux2/6
  Ground/1 -> Mux2/7
  Demux3/4 -> Mux2/4
  Demux3/2 -> Mux2/2
  Function Caller2/1 -> Demux4/1
  Data Store Read17/1 -> Function Caller2/1
  Demux3/1 -> Mux2/1
  Demux4/1 -> Mux2/5
  Function Caller1/1 -> Demux3/1
  Data Store Read12/1 -> Function Caller1/1
  Demux3/3 -> Mux2/3
  Mux2/1 -> data/1
  Constant/1 -> len/1

== system VCU_SW/logSignal/getListData/pageRawInput/getListDataII4 ==
  getListDataII4 : TriggerPort  TriggerType=function-call  IsSimulinkFunction=on  FunctionName=getListDataII4  FunctionVisibility=scoped  VariantControl=(inherit)
  Constant : Constant  Value=uint8(6)
  Data Store Read13 : DataStoreRead  DataStoreName=sTMSTempOutput
  Data Store Read18 : DataStoreRead  DataStoreName=sFirstGearVlvCur
  Demux5 : Demux
  Demux6 : Demux  Outputs=2
  Function Caller3 : FunctionCaller  FunctionPrototype=data = getListData.splitIntoTwoBytes(value)  InputArgumentSpecifications=<Enter example>  OutputArgumentSpecifications=<Enter example>
  Function Caller8 : FunctionCaller  FunctionPrototype=data = getListData.splitIntoFourBytes(value)  InputArgumentSpecifications=<Enter example>  OutputArgumentSpecifications=<Enter example>
  Ground1 : Ground
  Mux3 : Mux  Inputs=7
  data : ArgOut  DisableCoverage=on  OutDataTypeStr=uint8  PortDimensions=[1,7]  ArgumentName=data
  len : ArgOut  Port=2  OutDataTypeStr=uint8  ArgumentName=len
  wires:
  Function Caller8/1 -> Demux5/1
  Function Caller3/1 -> Demux6/1
  Data Store Read13/1 -> Function Caller8/1
  Demux6/2 -> Mux3/6
  Demux6/1 -> Mux3/5
  Data Store Read18/1 -> Function Caller3/1
  Demux5/2 -> Mux3/2
  Demux5/3 -> Mux3/3
  Demux5/4 -> Mux3/4
  Demux5/1 -> Mux3/1
  Ground1/1 -> Mux3/7
  Mux3/1 -> data/1
  Constant/1 -> len/1

== system VCU_SW/logSignal/getListData/pageRawInput/getListDataII5 ==
  getListDataII5 : TriggerPort  TriggerType=function-call  IsSimulinkFunction=on  FunctionName=getListDataII5  FunctionVisibility=scoped  VariantControl=(inherit)
  Constant : Constant  Value=uint8(6)
  Data Store Read19 : DataStoreRead  DataStoreName=sSecondGearVlvCur
  Data Store Read8 : DataStoreRead  DataStoreName=sFuseBoxTempSens1
  Demux7 : Demux
  Demux8 : Demux  Outputs=2
  Function Caller4 : FunctionCaller  FunctionPrototype=data = getListData.splitIntoTwoBytes(value)  InputArgumentSpecifications=<Enter example>  OutputArgumentSpecifications=<Enter example>
  Function Caller9 : FunctionCaller  FunctionPrototype=data = getListData.splitIntoFourBytes(value)  InputArgumentSpecifications=<Enter example>  OutputArgumentSpecifications=<Enter example>
  Ground2 : Ground
  Mux4 : Mux  Inputs=7
  data : ArgOut  DisableCoverage=on  OutDataTypeStr=uint8  PortDimensions=[1,7]  ArgumentName=data
  len : ArgOut  Port=2  OutDataTypeStr=uint8  ArgumentName=len
  wires:
  Function Caller9/1 -> Demux7/1
  Data Store Read19/1 -> Function Caller4/1
  Ground2/1 -> Mux4/7
  Demux8/2 -> Mux4/6
  Demux7/4 -> Mux4/4
  Demux7/1 -> Mux4/1
  Demux7/3 -> Mux4/3
  Function Caller4/1 -> Demux8/1
  Demux7/2 -> Mux4/2
  Demux8/1 -> Mux4/5
  Data Store Read8/1 -> Function Caller9/1
  Mux4/1 -> data/1
  Constant/1 -> len/1

== system VCU_SW/logSignal/getListData/pageRawInput/getListDataII6 ==
  getListDataII6 : TriggerPort  TriggerType=function-call  IsSimulinkFunction=on  FunctionName=getListDataII6  FunctionVisibility=scoped  VariantControl=(inherit)
  Constant : Constant  Value=uint8(6)
  Data Store Read20 : DataStoreRead  DataStoreName=sRemBrkVlvCur
  Data Store Read9 : DataStoreRead  DataStoreName=sFuseBoxTempSens2
  Demux10 : Demux  Outputs=2
  Demux9 : Demux
  Function Caller10 : FunctionCaller  FunctionPrototype=data = getListData.splitIntoFourBytes(value)  InputArgumentSpecifications=<Enter example>  OutputArgumentSpecifications=<Enter example>
  Function Caller5 : FunctionCaller  FunctionPrototype=data = getListData.splitIntoTwoBytes(value)  InputArgumentSpecifications=<Enter example>  OutputArgumentSpecifications=<Enter example>
  Ground3 : Ground
  Mux5 : Mux  Inputs=7
  data : ArgOut  DisableCoverage=on  OutDataTypeStr=uint8  PortDimensions=[1,7]  ArgumentName=data
  len : ArgOut  Port=2  OutDataTypeStr=uint8  ArgumentName=len
  wires:
  Function Caller10/1 -> Demux9/1
  Data Store Read20/1 -> Function Caller5/1
  Demux9/2 -> Mux5/2
  Demux9/3 -> Mux5/3
  Demux9/1 -> Mux5/1
  Demux10/2 -> Mux5/6
  Ground3/1 -> Mux5/7
  Function Caller5/1 -> Demux10/1
  Demux10/1 -> Mux5/5
  Data Store Read9/1 -> Function Caller10/1
  Demux9/4 -> Mux5/4
  Mux5/1 -> data/1
  Constant/1 -> len/1

== system VCU_SW/logSignal/getListData/pageRawInput/getListDataII7 ==
  getListDataII7 : TriggerPort  TriggerType=function-call  IsSimulinkFunction=on  FunctionName=getListDataII7  FunctionVisibility=scoped  VariantControl=(inherit)
  Constant : Constant  Value=uint8(6)
  Data Store Read15 : DataStoreRead  DataStoreName=sOutShaftFreq
  Data Store Read21 : DataStoreRead  DataStoreName=sTMSComprCur
  Demux11 : Demux  Outputs=2
  Demux12 : Demux
  Function Caller11 : FunctionCaller  FunctionPrototype=data = getListData.splitIntoFourBytes(value)  InputArgumentSpecifications=<Enter example>  OutputArgumentSpecifications=<Enter example>
  Function Caller7 : FunctionCaller  FunctionPrototype=data = getListData.splitIntoTwoBytes(value)  InputArgumentSpecifications=<Enter example>  OutputArgumentSpecifications=<Enter example>
  Ground4 : Ground
  Mux6 : Mux  Inputs=7
  data : ArgOut  DisableCoverage=on  OutDataTypeStr=uint8  PortDimensions=[1,7]  ArgumentName=data
  len : ArgOut  Port=2  OutDataTypeStr=uint8  ArgumentName=len
  wires:
  Function Caller7/1 -> Demux11/1
  Function Caller11/1 -> Demux12/1
  Demux11/2 -> Mux6/6
  Ground4/1 -> Mux6/7
  Demux12/4 -> Mux6/4
  Demux11/1 -> Mux6/5
  Demux12/2 -> Mux6/2
  Data Store Read21/1 -> Function Caller7/1
  Data Store Read15/1 -> Function Caller11/1
  Demux12/1 -> Mux6/1
  Demux12/3 -> Mux6/3
  Mux6/1 -> data/1
  Constant/1 -> len/1

== system VCU_SW/logSignal/getListData/pageRawInput/getListDataII8 ==
  getListDataII8 : TriggerPort  TriggerType=function-call  IsSimulinkFunction=on  FunctionName=getListDataII8  FunctionVisibility=scoped  VariantControl=(inherit)
  Constant : Constant  Value=uint8(6)
  Data Store Read16 : DataStoreRead  DataStoreName=sRingShaftFreq
  Data Store Read22 : DataStoreRead  DataStoreName=sCircPumpCur
  Demux13 : Demux  Outputs=2
  Demux14 : Demux
  Function Caller12 : FunctionCaller  FunctionPrototype=data = getListData.splitIntoFourBytes(value)  InputArgumentSpecifications=<Enter example>  OutputArgumentSpecifications=<Enter example>
  Function Caller6 : FunctionCaller  FunctionPrototype=data = getListData.splitIntoTwoBytes(value)  InputArgumentSpecifications=<Enter example>  OutputArgumentSpecifications=<Enter example>
  Ground5 : Ground
  Mux7 : Mux  Inputs=7
  data : ArgOut  DisableCoverage=on  OutDataTypeStr=uint8  PortDimensions=[1,7]  ArgumentName=data
  len : ArgOut  Port=2  OutDataTypeStr=uint8  ArgumentName=len
  wires:
  Function Caller6/1 -> Demux13/1
  Demux14/3 -> Mux7/3
  Data Store Read16/1 -> Function Caller12/1
  Demux13/1 -> Mux7/5
  Function Caller12/1 -> Demux14/1
  Data Store Read22/1 -> Function Caller6/1
  Demux14/2 -> Mux7/2
  Demux14/4 -> Mux7/4
  Demux13/2 -> Mux7/6
  Ground5/1 -> Mux7/7
  Demux14/1 -> Mux7/1
  Mux7/1 -> data/1
  Constant/1 -> len/1

== system VCU_SW/InputLayer/InputInterfaces/AnalogInput/AIProc1000msec/Filter ==
  note: Просто сделать статус загрязнено или не загрязнено
  1-D Lookup Table : Lookup_n-D  Commented=on  NumberOfTableDimensions=1  BreakpointsForDimension1=res_filter_X  Table=dP_filter_Y  InternalRulePriority=Speed  RndMeth=Simplest  InputSameDT=on
  Constant1 : Constant  Value=pMaxPressLoss
  Constant12 : Constant  Value=pFilterSensAccRes
  Constant2 : Constant  Value=pMinPressLoss
  Constant3 : Constant  Value=pPressLossTreshhold
  Constant8 : Constant  Value=pMaxFilterSensRes
  Constant9 : Constant  Value=pMinFilterSensRes
  Data Store Read11 : DataStoreRead  DataStoreName=InputInterfaceData  DataStoreElements=InputInterfaceData.AI.filterClogSens
  Data Store Write14 : DataStoreWrite  DataStoreName=InputFunctionsData  DataStoreElements=InputFunctionsData.filterPollutionState
  MATLAB Function1 : MATLAB Function  TreatAsAtomicUnit=on
  wires:
  Constant8/1 -> MATLAB Function1/1(maxRes)
  Constant9/1 -> MATLAB Function1/2(minRes)
  Constant12/1 -> MATLAB Function1/4(accuracyValue)
  Data Store Read11/1 -> MATLAB Function1/3(sensorValue)
  Constant1/1 -> MATLAB Function1/5(maxPress)
  Constant2/1 -> MATLAB Function1/6(minPress)
  MATLAB Function1/1(filterState) -> Data Store Write14/1
  Constant3/1 -> MATLAB Function1/7(Treshold)

== system VCU_SW/InputLayer/InputInterfaces/AnalogInput/AIProc1000msec/TemperatureValues ==
  Constant1 : Constant  Value=pMinTempValue
  Constant16 : Constant  Value=pMinTempValue
  Constant2 : Constant  Value=pMaxTempValue
  Constant28 : Constant  Value=pMaxTempValue
  Data Store Read1 : DataStoreRead  DataStoreName=InputInterfaceData  DataStoreElements=InputInterfaceData.AI.transPumpTempSens
  Data Store Read13 : DataStoreRead  DataStoreName=InputInterfaceData  DataStoreElements=InputInterfaceData.AI.hydMotTempSens
  Data Store Write1 : DataStoreWrite  DataStoreName=InputFunctionsData  DataStoreElements=InputFunctionsData.transPumpTemperature
  Data Store Write14 : DataStoreWrite  DataStoreName=InputFunctionsData  DataStoreElements=InputFunctionsData.hydMotTemperature
  Data Store Write2 : DataStoreWrite  DataStoreName=UDSStruct  DataStoreElements=UDSStruct.transPumpTempSens
  Data Store Write4 : DataStoreWrite  DataStoreName=UDSStruct  DataStoreElements=UDSStruct.hydMotTempSens
  Function Caller : FunctionCaller  FunctionPrototype=tempValue = TemperatureValues.calcCurPressSens(sensValue,tempMax,tempMin)  InputArgumentSpecifications=<Enter example>  OutputArgumentSpecifications=<Enter example>
  Function Caller1 : FunctionCaller  FunctionPrototype=tempValue = TemperatureValues.calcCurPressSens(sensValue,tempMax,tempMin)  InputArgumentSpecifications=<Enter example>  OutputArgumentSpecifications=<Enter example>
  calcCurPressSensVal : Subsystem  TreatAsAtomicUnit=on
  calcFuseTemp : Subsystem  Commented=on  TreatAsAtomicUnit=on
  calcTMSTemp : Subsystem  Commented=on  TreatAsAtomicUnit=on
  wires:
  Function Caller1/1 -> Data Store Write1/1, Data Store Write2/1
  Function Caller/1 -> Data Store Write14/1, Data Store Write4/1
  Constant16/1 -> Function Caller/3
  Constant28/1 -> Function Caller/2
  Data Store Read13/1 -> Function Caller/1
  Data Store Read1/1 -> Function Caller1/1
  Constant2/1 -> Function Caller1/2
  Constant1/1 -> Function Caller1/3

== system VCU_SW/InputLayer/InputInterfaces/AnalogInput/AIProc100msec/GenWorkSig ==
  Data Store Read : DataStoreRead  DataStoreName=InputInterfaceData  DataStoreElements=InputInterfaceData.AI.upperGenWorkSig
  Data Store Read1 : DataStoreRead  DataStoreName=InputInterfaceData  DataStoreElements=InputInterfaceData.AI.lowerGenWorkSig
  Data Store Write : DataStoreWrite  DataStoreName=InputFunctionsData  DataStoreElements=InputFunctionsData.upperGenWorkSignal
  Data Store Write1 : DataStoreWrite  DataStoreName=InputFunctionsData  DataStoreElements=InputFunctionsData.lowerGenWorkSignal
  Function Caller : FunctionCaller  FunctionPrototype=finalState = voltageAIConv(Volt)  InputArgumentSpecifications=<Enter example>  OutputArgumentSpecifications=<Enter example>
  Function Caller1 : FunctionCaller  FunctionPrototype=finalState = voltageAIConv(Volt)  InputArgumentSpecifications=<Enter example>  OutputArgumentSpecifications=<Enter example>
  wires:
  Data Store Read/1 -> Function Caller/1
  Data Store Read1/1 -> Function Caller1/1
  Function Caller/1 -> Data Store Write/1
  Function Caller1/1 -> Data Store Write1/1

== system VCU_SW/InputLayer/InputInterfaces/AnalogInput/AIProc100msec/PressureValues ==
  Constant10 : Constant  Value=pMaxPressValue
  Constant11 : Constant  Value=pMaxPressValue
  Constant13 : Constant  Value=pMinPressValue
  Constant14 : Constant  Value=pMinPressValue
  Constant15 : Constant  Value=pMinPressValue
  Constant24 : Constant  Value=pMaxPressValueParkDrain
  Data Store Read10 : DataStoreRead  DataStoreName=InputInterfaceData  DataStoreElements=InputInterfaceData.AI.brkSupplyFrontPressSens
  Data Store Read11 : DataStoreRead  DataStoreName=InputInterfaceData  DataStoreElements=InputInterfaceData.AI.brkSupplyParkPressSens
  Data Store Read9 : DataStoreRead  DataStoreName=InputInterfaceData  DataStoreElements=InputInterfaceData.AI.brkSupplyRearPressSens
  Data Store Write10 : DataStoreWrite  DataStoreName=InputFunctionsData  DataStoreElements=InputFunctionsData.supplyRearBrakePressure
  Data Store Write11 : DataStoreWrite  DataStoreName=InputFunctionsData  DataStoreElements=InputFunctionsData.supplyFrontBrakePressure
  Data Store Write12 : DataStoreWrite  DataStoreName=InputFunctionsData  DataStoreElements=InputFunctionsData.supplyParkBrakePressure
  Data Store Write3 : DataStoreWrite  DataStoreName=UDSStruct  DataStoreElements=UDSStruct.brkSupplyRearPressSens
  Data Store Write4 : DataStoreWrite  DataStoreName=UDSStruct  DataStoreElements=UDSStruct.brkSupplyFrontPressSens
  Data Store Write5 : DataStoreWrite  DataStoreName=UDSStruct  DataStoreElements=UDSStruct.brkSupplyParkPressSens
  Data Type Conversion : DataTypeConversion  OutDataTypeStr=uint16
  Data Type Conversion1 : DataTypeConversion  OutDataTypeStr=uint16
  Data Type Conversion2 : DataTypeConversion  OutDataTypeStr=uint16
  Function Caller : FunctionCaller  FunctionPrototype=pressValue = PressureValues.calcCurPressSens(sensValue,pressMax,pressMin)  InputArgumentSpecifications=<Enter example>  OutputArgumentSpecifications=<Enter example>
  Function Caller11 : FunctionCaller  FunctionPrototype=pressValue = PressureValues.calcCurPressSens(sensValue,pressMax,pressMin)  InputArgumentSpecifications=<Enter example>  OutputArgumentSpecifications=<Enter example>
  Function Caller8 : FunctionCaller  FunctionPrototype=pressValue = PressureValues.calcCurPressSens(sensValue,pressMax,pressMin)  InputArgumentSpecifications=<Enter example>  OutputArgumentSpecifications=<Enter example>
  Gain : Gain  Gain=1/1000  OutDataTypeStr=Inherit: Same as input
  Gain1 : Gain  Gain=1/1000  OutDataTypeStr=Inherit: Same as input
  Gain2 : Gain  Gain=1/1000  OutDataTypeStr=Inherit: Same as input
  calcCurPressSensVal : Subsystem  TreatAsAtomicUnit=on
  wires:
  Function Caller11/1 -> Gain2/1, Data Store Write12/1
  Function Caller8/1 -> Gain1/1, Data Store Write11/1
  Function Caller/1 -> Data Store Write10/1, Gain/1
  Constant15/1 -> Function Caller11/3
  Data Store Read11/1 -> Function Caller11/1
  Constant24/1 -> Function Caller11/2
  Constant14/1 -> Function Caller8/3
  Data Store Read10/1 -> Function Caller8/1
  Constant11/1 -> Function Caller8/2
  Data Store Read9/1 -> Function Caller/1
  Constant10/1 -> Function Caller/2
  Constant13/1 -> Function Caller/3
  Gain/1 -> Data Type Conversion/1
  Data Type Conversion/1 -> Data Store Write3/1
  Gain1/1 -> Data Type Conversion1/1
  Data Type Conversion1/1 -> Data Store Write4/1
  Gain2/1 -> Data Type Conversion2/1
  Data Type Conversion2/1 -> Data Store Write5/1
